simulink model "aerodynamics_v2"  (R2025b)
settings: Solver=VariableStepAuto  StartTime=0.0  StopTime=50  RelTol=1e-3
libraries: simulink x1
settings Model: Creator=rosette-nebula  LastModifiedBy=rosette-nebula

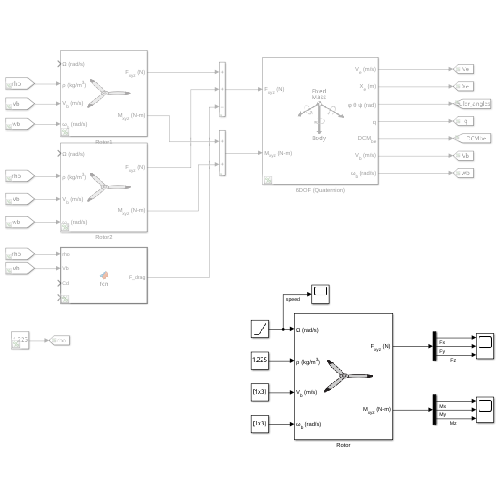
[thumbnail: Simulink's stored preview of the top-level diagram]
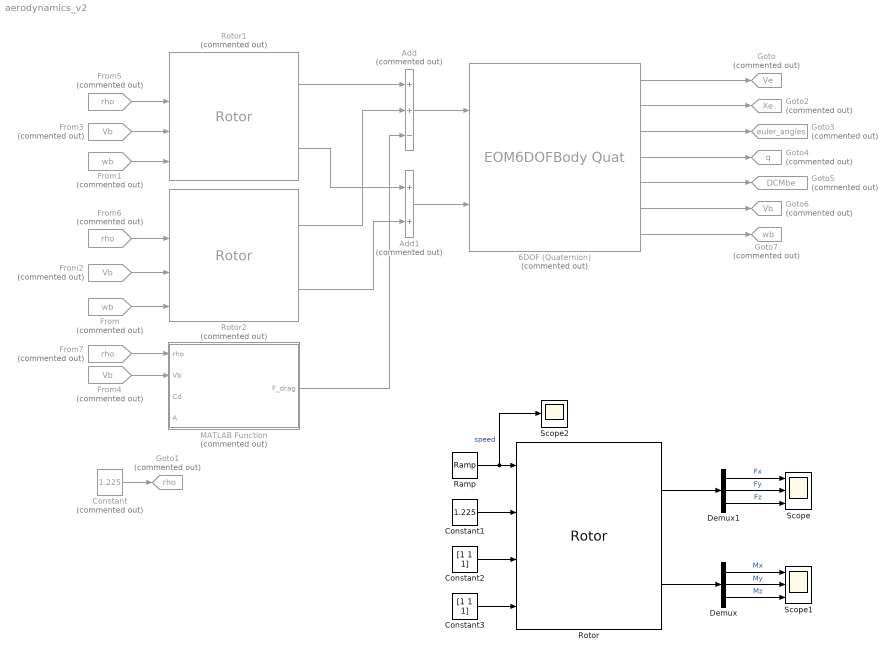
== system aerodynamics_v2 ==
  6DOF (Quaternion) : EOM6DOFBodyQuat  Commented=on
  Add : Sum  Commented=on  Inputs=++-
  Add1 : Sum  Commented=on
  Constant : Constant  Commented=on  Value=1.225
  Constant1 : Constant  Value=1.225
  Constant2 : Constant  Value=[1 1 1]
  Constant3 : Constant  Value=[1 1 1]
  Demux : Demux  Outputs=3
  Demux1 : Demux  Outputs=3
  From : From  Commented=on  GotoTag=wb  TagVisibility=global
  From1 : From  Commented=on  GotoTag=wb  TagVisibility=global
  From2 : From  Commented=on  GotoTag=Vb  TagVisibility=global
  From3 : From  Commented=on  GotoTag=Vb  TagVisibility=global
  From4 : From  Commented=on  GotoTag=Vb  TagVisibility=global
  From5 : From  Commented=on  GotoTag=rho  TagVisibility=global
  From6 : From  Commented=on  GotoTag=rho  TagVisibility=global
  From7 : From  Commented=on  GotoTag=rho  TagVisibility=global
  Goto : Goto  Commented=on  GotoTag=Ve  TagVisibility=global
  Goto1 : Goto  Commented=on  GotoTag=rho  TagVisibility=global
  Goto2 : Goto  Commented=on  GotoTag=Xe  TagVisibility=global
  Goto3 : Goto  Commented=on  GotoTag=euler_angles  TagVisibility=global
  Goto4 : Goto  Commented=on  GotoTag=q  TagVisibility=global
  Goto5 : Goto  Commented=on  GotoTag=DCMbe  TagVisibility=global
  Goto6 : Goto  Commented=on  GotoTag=Vb  TagVisibility=global
  Goto7 : Goto  Commented=on  GotoTag=wb  TagVisibility=global
  MATLAB Function : MATLAB Function  Commented=on  TreatAsAtomicUnit=on
  Ramp : simulink/Sources/Ramp  slope=-1000  start=0  InitialOutput=0
  Rotor : Rotor  modelMode=With flap effects  radius=0.100214  chord=0.094248  clalpha=2*pi
  Rotor1 : Rotor  Commented=on  modelMode=With flap effects  radius=0.204/2
  Rotor2 : Rotor  Commented=on  modelMode=With flap effects
  Scope : Scope  NumInputPorts=3
      settings: ActiveDisplayYMinimum=-0.799625211243045  ActiveDisplayYMaximum=7.1966269011874067
  Scope1 : Scope  NumInputPorts=3
      settings: ActiveDisplayYMinimum=-1  ActiveDisplayYMaximum=1
  Scope2 : Scope
      settings: ActiveDisplayYMinimum=-56250  ActiveDisplayYMaximum=6249.9999999999982  DataLoggingVariableName=ScopeData2
  wires:
  6DOF (Quaternion)/4 -> Goto4/1
  6DOF (Quaternion)/2 -> Goto2/1
  6DOF (Quaternion)/1 -> Goto/1
  6DOF (Quaternion)/3 -> Goto3/1
  6DOF (Quaternion)/5 -> Goto5/1
  6DOF (Quaternion)/6 -> Goto6/1
  6DOF (Quaternion)/7 -> Goto7/1
  Rotor1/1 -> Add/1
  Rotor2/1 -> Add/2
  MATLAB Function/1(F_drag) -> Add/3
  Add/1 -> 6DOF (Quaternion)/1
  From/1 -> Rotor2/4
  From1/1 -> Rotor1/4
  From2/1 -> Rotor2/3
  From3/1 -> Rotor1/3
  Add1/1 -> 6DOF (Quaternion)/2
  Rotor2/2 -> Add1/2
  Rotor1/2 -> Add1/1
  From4/1 -> MATLAB Function/2(Vb)
  Constant/1 -> Goto1/1
  From5/1 -> Rotor1/2
  From6/1 -> Rotor2/2
  From7/1 -> MATLAB Function/1(rho)
  Rotor/1 -> Demux1/1
  Rotor/2 -> Demux/1
  Demux1/3 -> Scope/3  "Fz"
  Demux/3 -> Scope1/3  "Mz"
  Constant1/1 -> Rotor/2
  Constant2/1 -> Rotor/3
  Constant3/1 -> Rotor/4
  Ramp/1 -> Scope2/1, Rotor/1  "speed"
  Demux1/1 -> Scope/1  "Fx"
  Demux1/2 -> Scope/2  "Fy"
  Demux/1 -> Scope1/1  "Mx"
  Demux/2 -> Scope1/2  "My"

== matlab function aerodynamics_v2/MATLAB Function ==
  data: rho input; F_drag output; Vb input; Cd input; A input
function F_drag = fcn(rho, Vb, Cd, A)

F_drag = -0.5*rho*dot(Vb,Vb)*Cd*A * (Vb/norm(Vb));
